simulink model "calibration"  (R2018a)
settings: Solver=VariableStepAuto  StartTime=0.0  StopTime=40  RelTol=1e-3
values from neighbouring files (symbols this model uses):
  aubr = -8:0.05:5    [generate_calibration.m]
  tablebr = zeros(length(vubr),length(aubr))    [generate_calibration.m]
  vubr = 0:0.05:50    [generate_calibration.m]
  x = x-0.1    (= -0.1)    [brake_calibration.m]    (also in thr_calibration.m = 0.05)
libraries: Solver_SF x1, simulink x1
settings Model: Creator=wwcong  LastModifiedBy=wwcong

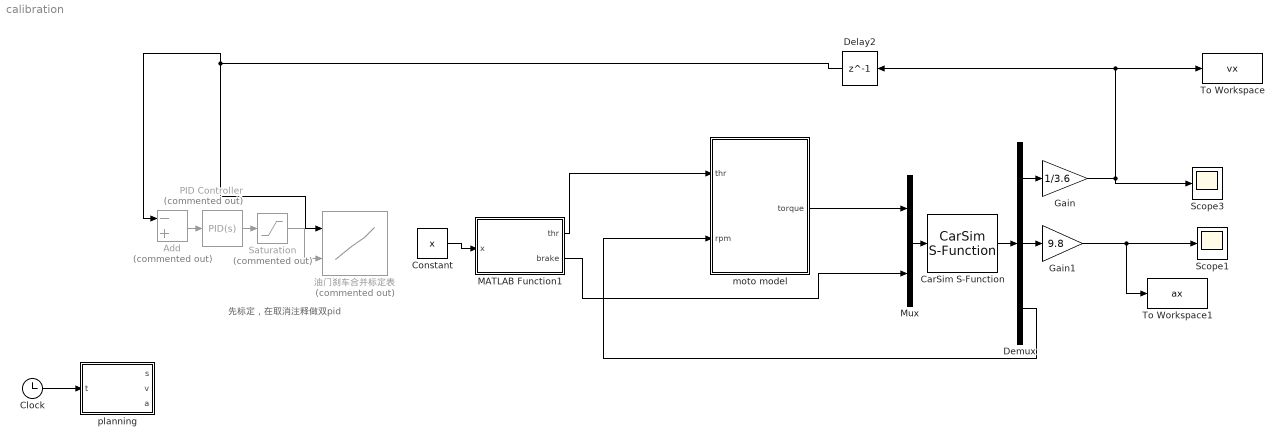
== system calibration ==
  note: 先标定，在取消注释做双pid
  Add : Sum  Commented=on  Inputs=-+
  CarSim S-Function : Solver_SF/CarSim S-Function  Priority=1  SIMFILE=simfile.sim
  Clock : Clock
  Constant : Constant  Value=x
  Delay2 : Delay  DelayLength=1
  Demux : Demux  Outputs=3
  Gain : Gain  Gain=1/3.6
  Gain1 : Gain  Gain=9.8
  MATLAB Function1 : MATLAB Function  TreatAsAtomicUnit=on
  Mux : Mux  Inputs=2
  PID Controller : simulink/Continuous/PID Controller  Commented=on  Controller=PID  TimeDomain=Continuous-time  SampleTime=-1  IntegratorMethod=Forward Euler  FilterMethod=Forward Euler  Form=Parallel  UseFilter=on  ControllerParametersSource=internal  P=6  I=0  D=0.1  N=30  InitialConditionSource=internal  InitialConditionForIntegrator=0  InitialConditionForFilter=0  ExternalReset=none  LimitOutput=off  UpperSaturationLimit=inf  LowerSaturationLimit=-inf  LinearizeAsGain=on  AntiWindupMode=none  Kb=1  TrackingMode=off  Kt=1  PParamMin=[]  PParamMax=[]  IParamMin=[]  IParamMax=[]  DParamMin=[]  DParamMax=[]  NParamMin=[]  NParamMax=[]  KbParamMin=[]  KbParamMax=[]  KtParamMin=[]  KtParamMax=[]  POutMin=[]  POutMax=[]  IOutMin=[]  IOutMax=[]  DOutMin=[]  DOutMax=[]  NOutMin=[]  NOutMax=[]  KbOutMin=[]  KbOutMax=[]  KtOutMin=[]  KtOutMax=[]  IntegratorOutMin=[]  IntegratorOutMax=[]  FilterOutMin=[]  FilterOutMax=[]  SumOutMin=[]  SumOutMax=[]  SumI1OutMin=[]  SumI1OutMax=[]  SumI2OutMin=[]  SumI2OutMax=[]  SumI3OutMin=[]  SumI3OutMax=[]  SumDOutMin=[]  SumDOutMax=[]  SaturationOutMin=[]  SaturationOutMax=[]  IntegratorContinuousStateAttributes=''  IntegratorStateMustResolveToSignalObject=off  IntegratorRTWStateStorageClass=Auto  FilterContinuousStateAttributes=''  FilterStateMustResolveToSignalObject=off  FilterRTWStateStorageClass=Auto  DifferentiatorICPrevScaledInput=0  DifferentiatorOutMin=[]  DifferentiatorOutMax=[]  FilterDiffOutCoefMin=[]  FilterDiffOutCoefMax=[]  SumDenOutMin=[]  SumDenOutMax=[]  SumNumOutMin=[]  SumNumOutMax=[]  ReciprocalOutMin=[]  ReciprocalOutMax=[]  DivideOutMin=[]  DivideOutMax=[]  TunerSelectOption=Transfer Function Based (PID Tuner App)
  Saturation : Saturate  Commented=on  UpperLimit=5  LowerLimit=-8
  Scope1 : Scope
  Scope3 : Scope
  To Workspace : ToWorkspace  VariableName=vx  SaveFormat=Timeseries  SampleTime=0.15
  To Workspace1 : ToWorkspace  VariableName=ax  SaveFormat=Timeseries  SampleTime=0.15
  moto model : MATLAB Function  TreatAsAtomicUnit=on
  planning : MATLAB Function  TreatAsAtomicUnit=on
  油门刹车合并标定表 : Lookup_n-D  Commented=on  BreakpointsForDimension1=vubr  BreakpointsForDimension2=aubr  Table=tablebr  InternalRulePriority=Speed  RndMeth=Simplest  InputSameDT=on
  wires:
  Mux/1 -> CarSim S-Function/1
  CarSim S-Function/1 -> Demux/1
  Demux/1 -> Gain/1
  Demux/2 -> Gain1/1
  Gain1/1 -> To Workspace1/1, Scope1/1
  Gain/1 -> Delay2/1, To Workspace/1, Scope3/1
  Add/1 -> PID Controller/1
  PID Controller/1 -> Saturation/1
  moto model/1(torque) -> Mux/1
  MATLAB Function1/2(brake) -> Mux/2
  Delay2/1 -> Add/1, 油门刹车合并标定表/1
  Demux/3 -> moto model/2(rpm)
  MATLAB Function1/1(thr) -> moto model/1(thr)
  Saturation/1 -> 油门刹车合并标定表/2
  Constant/1 -> MATLAB Function1/1(x)
  Clock/1 -> planning/1(t)

== matlab function calibration/MATLAB Function1 ==
  data: x input; thr output; brake output
function [thr,brake] = fcn(x)
    %正数代表油门，负数代表刹车
    %不允许同时踩油门和刹车
    if x>=0
        thr=x;
        brake=0;
    else
        thr=0;
        brake=-x;
    end

== matlab function calibration/moto model ==
  data: thr input; torque output; rpm input
function torque = fcn(thr,rpm)
Tmax=380*thr;
    if (rpm<=4523)
        torque=Tmax;
    else
        torque=Tmax*4523/rpm;
    end
end

== matlab function calibration/planning ==
  data: t input; s output; v output; a output
function [s,v,a] = fcn(t)
if t<10
    s=0.1*t^3/3;
    v=0.1*t^2;
    a=0.2*t;
else
    a=2-0.1*(t-10);
    v=2*t-0.05*(t-10)^2-10;
    s=t^2-0.05*(t-10)^3/3-10*t+100/3;
end
